simulink model "motor_pos_ctrl"  (R2023b)
settings: Solver=VariableStepAuto  StartTime=0.0  StopTime=1  RelTol=1e-3
InitFcn:
  | %%%%%%%%%%%%%%%%%%%%%%%%%%%%%%%%%%%%%%%%%%%%%%%%%
  | %motor parameters
  | %we dont know these yet
  | J = 1e-6; %intertia [kg * m^2]
  | Bm = 1e-6; %kinetic friction [N * m * s]
  | 
  | %from motor datasheet
  | Km = 0.011; %motor constant (back emf constant = torque constant)
  | Rw = 1.17; %motor electric resistance in ohms
  | Lw = 0.58E-3; %motor inductance in ohms
  | 
  | sample_time_s = 1e-3;
libraries: slpidlib x2
settings Model: Creator=you29  LastModifiedBy=you29

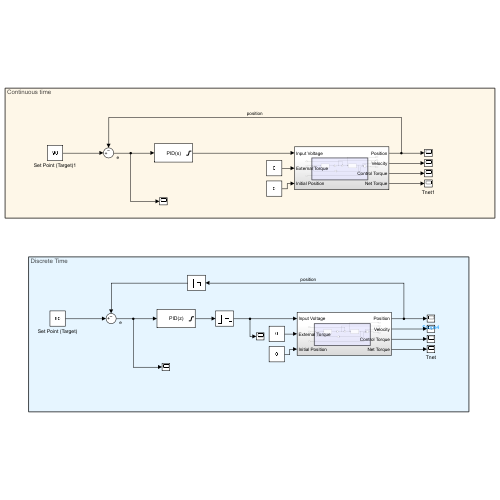
[thumbnail: Simulink's stored preview of the top-level diagram]
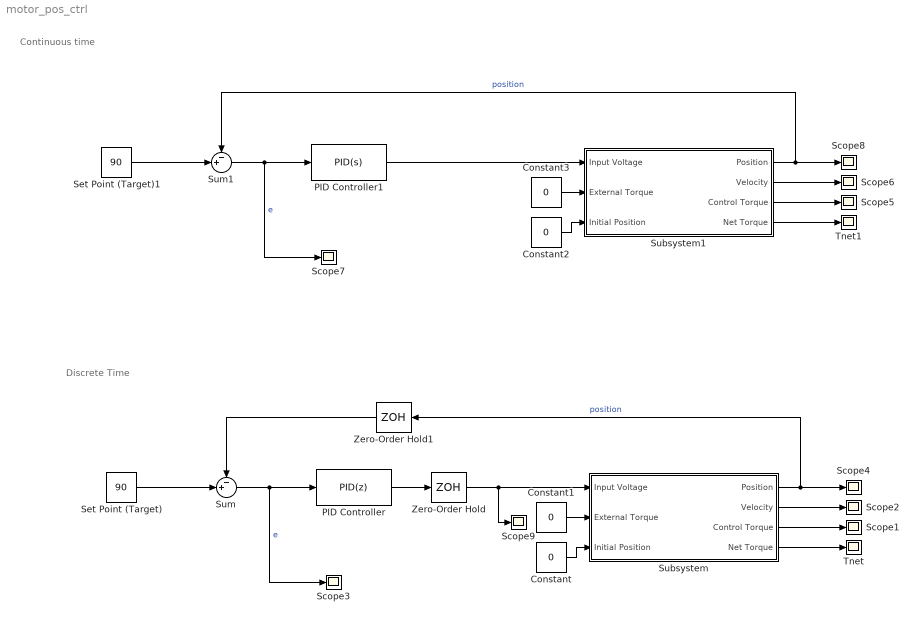
== system motor_pos_ctrl ==
  note: Continuous time
  note: Discrete Time
  Constant{,1..3} (4 alike) : Constant  Value=0
  PID Controller : slpidlib/PID Controller  Controller=PID  Form=Parallel  TimeDomain=Discrete-time  UseExternalTs=off  SampleTime=-1  IntegratorMethod=Forward Euler  FilterMethod=Forward Euler  ControllerParametersSource=internal  P=2.78055118948692  I=5  UseKiTs=off  D=0.0179888997776462  N=1  UseFilter=on  TunerSelectOption=Transfer Function Based (PID Tuner App)  InitialConditionSource=internal  InitialConditionForIntegrator=0  InitialConditionForFilter=0  DifferentiatorICPrevScaledInput=0  ExternalReset=none  TrackingMode=off  Kt=1  LimitOutput=on  SatLimitsSource=internal  UpperSaturationLimit=12  LowerSaturationLimit=-12  LinearizeAsGain=on  AntiWindupMode=none  Kb=1  LimitIntegrator=off  UpperIntegratorSaturationLimit=inf  LowerIntegratorSaturationLimit=-inf  POutMin=[]  POutMax=[]  IOutMin=[]  IOutMax=[]  DOutMin=[]  DOutMax=[]  NOutMin=[]  NOutMax=[]  SumOutMin=[]  SumOutMax=[]  SaturationOutMin=[]  SaturationOutMax=[]  PParamMin=[]  PParamMax=[]  IParamMin=[]  IParamMax=[]  DParamMin=[]  DParamMax=[]  NParamMin=[]  NParamMax=[]  KbParamMin=[]  KbParamMax=[]  KtParamMin=[]  KtParamMax=[]  KbOutMin=[]  KbOutMax=[]  KtOutMin=[]  KtOutMax=[]  IntegratorOutMin=[]  IntegratorOutMax=[]  FilterOutMin=[]  FilterOutMax=[]  SumI1OutMin=[]  SumI1OutMax=[]  SumI2OutMin=[]  SumI2OutMax=[]  SumI3OutMin=[]  SumI3OutMax=[]  SumI4OutMin=[]  SumI4OutMax=[]  SumDOutMin=[]  SumDOutMax=[]  DifferentiatorOutMin=[]  DifferentiatorOutMax=[]  FilterDiffOutCoefMin=[]  FilterDiffOutCoefMax=[]  ReciprocalOutMin=[]  ReciprocalOutMax=[]  SumDenOutMin=[]  SumDenOutMax=[]  SumNumOutMin=[]  SumNumOutMax=[]  DivideOutMin=[]  DivideOutMax=[]  UdiffTsProdOutMin=[]  UdiffTsProdOutMax=[]  NTsProdOutMin=[]  NTsProdOutMax=[]  UintegralTsProdOutMin=[]  UintegralTsProdOutMax=[]  UngainTsProdOutMin=[]  UngainTsProdOutMax=[]  ClampingZeroOutDataTypeStr=Inherit: Inherit via back propagation  ClampingZeroOutMin=[]  ClampingZeroOutMax=[]  FilterDenConstantOutDataTypeStr=Inherit: Inherit via back propagation  FilterDenConstantOutMin=[]  FilterDenConstantOutMax=[]  PCopyOutDataTypeStr=Inherit: Inherit via back propagation  PCopyOutMin=[]  PCopyOutMax=[]  NCopyOutDataTypeStr=Inherit: Inherit via back propagation  NCopyOutMin=[]  NCopyOutMax=[]  IntegratorContinuousStateAttributes=''  IntegratorStateMustResolveToSignalObject=off  IntegratorRTWStateStorageClass=Auto  FilterContinuousStateAttributes=''  FilterStateMustResolveToSignalObject=off  FilterRTWStateStorageClass=Auto  ParallelPVariant=InternalParameters  IdealPVariant=Disabled  IVariant=InternalParameters  DVariant=InternalParameters  IntegratorVariant=Discrete  SatVariant=Enabled  AWVariant=Passthrough  PCopyVariant=Disabled  TRVariant=Disabled  FdbkBlocksVariant=Forward  IdealPFdbkVariant=Disabled  SatFdbkVariant=Disabled  DerivativeFilterVariant=ForwardEulerFilter  NVariant=InternalParameters  NCopyVariant=Disabled  FilterICVariant=InternalICsFilter  IntegratorICVariant=InternalICs  ExternalResetVariant=Disabled  TRSumVariant=Passthrough  SumFdbkVariant=Disabled  SumVariant=Sum_PID  TsampFilterVariant=InternalTs  TsampNgainVariant=Passthrough  TsampIntegralVariant=Disabled_SignalSpec  ExternalSaturationOutDataTypeStr=Inherit: Same as second input
  PID Controller1 : slpidlib/PID Controller  Controller=PID  Form=Parallel  TimeDomain=Continuous-time  UseExternalTs=off  SampleTime=-1  IntegratorMethod=Forward Euler  FilterMethod=Forward Euler  ControllerParametersSource=internal  P=2.78055118948692  I=5  UseKiTs=off  D=0.0179888997776462  N=1  UseFilter=on  TunerSelectOption=Transfer Function Based (PID Tuner App)  InitialConditionSource=internal  InitialConditionForIntegrator=0  InitialConditionForFilter=0  DifferentiatorICPrevScaledInput=0  ExternalReset=none  TrackingMode=off  Kt=1  LimitOutput=on  SatLimitsSource=internal  UpperSaturationLimit=12  LowerSaturationLimit=-12  LinearizeAsGain=on  AntiWindupMode=none  Kb=1  LimitIntegrator=off  UpperIntegratorSaturationLimit=inf  LowerIntegratorSaturationLimit=-inf  POutMin=[]  POutMax=[]  IOutMin=[]  IOutMax=[]  DOutMin=[]  DOutMax=[]  NOutMin=[]  NOutMax=[]  SumOutMin=[]  SumOutMax=[]  SaturationOutMin=[]  SaturationOutMax=[]  PParamMin=[]  PParamMax=[]  IParamMin=[]  IParamMax=[]  DParamMin=[]  DParamMax=[]  NParamMin=[]  NParamMax=[]  KbParamMin=[]  KbParamMax=[]  KtParamMin=[]  KtParamMax=[]  KbOutMin=[]  KbOutMax=[]  KtOutMin=[]  KtOutMax=[]  IntegratorOutMin=[]  IntegratorOutMax=[]  FilterOutMin=[]  FilterOutMax=[]  SumI1OutMin=[]  SumI1OutMax=[]  SumI2OutMin=[]  SumI2OutMax=[]  SumI3OutMin=[]  SumI3OutMax=[]  SumI4OutMin=[]  SumI4OutMax=[]  SumDOutMin=[]  SumDOutMax=[]  DifferentiatorOutMin=[]  DifferentiatorOutMax=[]  FilterDiffOutCoefMin=[]  FilterDiffOutCoefMax=[]  ReciprocalOutMin=[]  ReciprocalOutMax=[]  SumDenOutMin=[]  SumDenOutMax=[]  SumNumOutMin=[]  SumNumOutMax=[]  DivideOutMin=[]  DivideOutMax=[]  UdiffTsProdOutMin=[]  UdiffTsProdOutMax=[]  NTsProdOutMin=[]  NTsProdOutMax=[]  UintegralTsProdOutMin=[]  UintegralTsProdOutMax=[]  UngainTsProdOutMin=[]  UngainTsProdOutMax=[]  ClampingZeroOutDataTypeStr=Inherit: Inherit via back propagation  ClampingZeroOutMin=[]  ClampingZeroOutMax=[]  FilterDenConstantOutDataTypeStr=Inherit: Inherit via back propagation  FilterDenConstantOutMin=[]  FilterDenConstantOutMax=[]  PCopyOutDataTypeStr=Inherit: Inherit via back propagation  PCopyOutMin=[]  PCopyOutMax=[]  NCopyOutDataTypeStr=Inherit: Inherit via back propagation  NCopyOutMin=[]  NCopyOutMax=[]  IntegratorContinuousStateAttributes=''  IntegratorStateMustResolveToSignalObject=off  IntegratorRTWStateStorageClass=Auto  FilterContinuousStateAttributes=''  FilterStateMustResolveToSignalObject=off  FilterRTWStateStorageClass=Auto  ParallelPVariant=InternalParameters  IdealPVariant=Disabled  IVariant=InternalParameters  DVariant=InternalParameters  IntegratorVariant=Continuous  SatVariant=Enabled  AWVariant=Passthrough  PCopyVariant=Disabled  TRVariant=Disabled  FdbkBlocksVariant=Forward  IdealPFdbkVariant=Disabled  SatFdbkVariant=Disabled  DerivativeFilterVariant=ContFilter  NVariant=InternalParameters  NCopyVariant=Disabled  FilterICVariant=InternalICsFilter  IntegratorICVariant=InternalICs  ExternalResetVariant=Disabled  TRSumVariant=Passthrough  SumFdbkVariant=Disabled  SumVariant=Sum_PID  TsampFilterVariant=InternalTs  TsampNgainVariant=Passthrough  TsampIntegralVariant=Disabled_SignalSpec  ExternalSaturationOutDataTypeStr=Inherit: Same as second input
  Scope{1..9} (9 alike) : Scope
  Set Point (Target) : Constant  Value=90
  Set Point (Target)1 : Constant  Value=90
  Subsystem : Subsystem
  Subsystem1 : Subsystem
  Sum : Sum  Inputs=-+|
  Sum1 : Sum  Inputs=-+|
  Tnet : Scope
  Tnet1 : Scope
  Zero-Order Hold : ZeroOrderHold  SampleTime=sample_time_s
  Zero-Order Hold1 : ZeroOrderHold  SampleTime=sample_time_s
  wires:
  Constant/1 -> Subsystem/3(Initial Position)
  Subsystem/1(Position) -> Scope4/1, Zero-Order Hold1/1  "position"
  Set Point (Target)/1 -> Sum/2
  Constant1/1 -> Subsystem/2(External Torque)
  Subsystem/4(Net Torque) -> Tnet/1
  Subsystem/3(Control Torque) -> Scope1/1
  Subsystem/2(Velocity) -> Scope2/1
  Sum/1 -> Scope3/1, PID Controller/1  "e"
  PID Controller/1 -> Zero-Order Hold/1
  Zero-Order Hold/1 -> Scope9/1, Subsystem/1(Input Voltage)
  Zero-Order Hold1/1 -> Sum/1
  PID Controller1/1 -> Subsystem1/1(Input Voltage)
  Sum1/1 -> Scope7/1, PID Controller1/1  "e"
  Subsystem1/3(Control Torque) -> Scope5/1
  Subsystem1/4(Net Torque) -> Tnet1/1
  Constant3/1 -> Subsystem1/2(External Torque)
  Set Point (Target)1/1 -> Sum1/2
  Subsystem1/1(Position) -> Sum1/1, Scope8/1  "position"
  Constant2/1 -> Subsystem1/3(Initial Position)
  Subsystem1/2(Velocity) -> Scope6/1

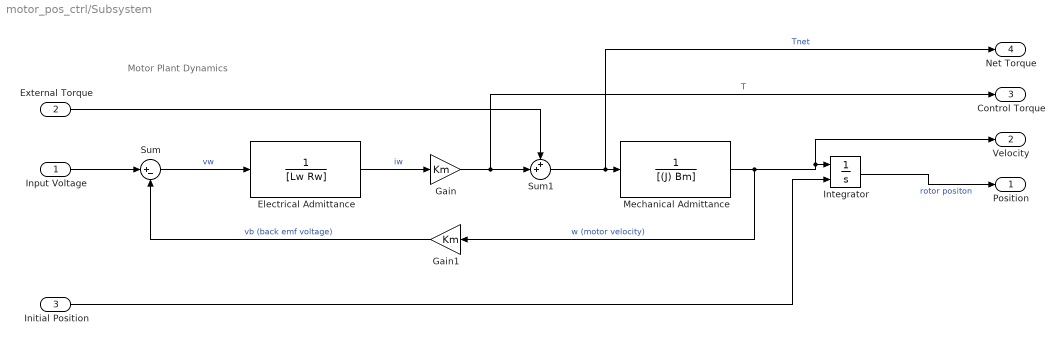
== system motor_pos_ctrl/Subsystem ==
  note: Motor Plant Dynamics
  Input Voltage : Inport
  External Torque : Inport  Port=2
  Initial Position : Inport  Port=3
  Electrical Admittance : TransferFcn  Denominator=[Lw Rw]
  Gain : Gain  Gain=Km
  Gain1 : Gain  Gain=Km
  Integrator : Integrator  InitialConditionSource=external
  Mechanical Admittance : TransferFcn  Denominator=[(J) Bm]
  Sum : Sum  Inputs=|+-
  Sum1 : Sum  Inputs=++|
  Position : Outport
  Velocity : Outport  Port=2
  Control Torque : Outport  Port=3
  Net Torque : Outport  Port=4
  wires:
  Input Voltage/1 -> Sum/1
  Mechanical Admittance/1 -> Velocity/1, Integrator/1, Gain1/1  "w (motor velocity)"
  Gain1/1 -> Sum/2  "vb (back emf voltage)"
  Integrator/1 -> Position/1  "rotor positon"
  Gain/1 -> Control Torque/1, Sum1/2  "T"
  Electrical Admittance/1 -> Gain/1  "iw"
  Sum/1 -> Electrical Admittance/1  "vw"
  Sum1/1 -> Net Torque/1, Mechanical Admittance/1  "Tnet"
  External Torque/1 -> Sum1/1
  Initial Position/1 -> Integrator/2

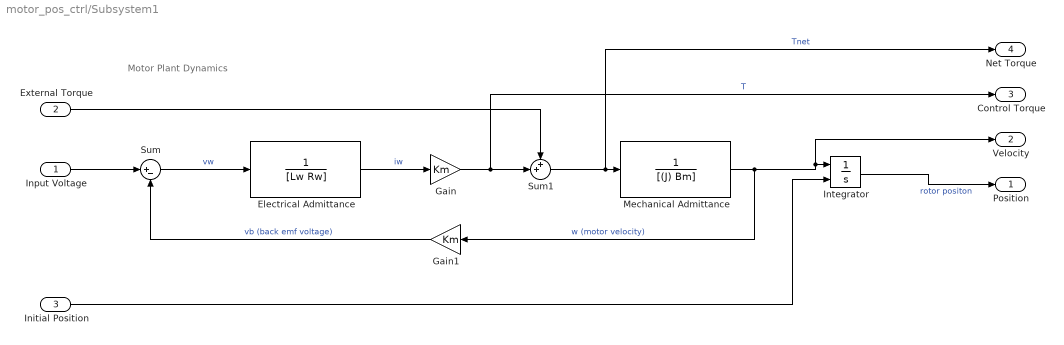
== system motor_pos_ctrl/Subsystem1 ==
  note: Motor Plant Dynamics
  Input Voltage : Inport
  External Torque : Inport  Port=2
  Initial Position : Inport  Port=3
  Electrical Admittance : TransferFcn  Denominator=[Lw Rw]
  Gain : Gain  Gain=Km
  Gain1 : Gain  Gain=Km
  Integrator : Integrator  InitialConditionSource=external
  Mechanical Admittance : TransferFcn  Denominator=[(J) Bm]
  Sum : Sum  Inputs=|+-
  Sum1 : Sum  Inputs=++|
  Position : Outport
  Velocity : Outport  Port=2
  Control Torque : Outport  Port=3
  Net Torque : Outport  Port=4
  wires:
  Input Voltage/1 -> Sum/1
  Mechanical Admittance/1 -> Velocity/1, Integrator/1, Gain1/1  "w (motor velocity)"
  Gain1/1 -> Sum/2  "vb (back emf voltage)"
  Integrator/1 -> Position/1  "rotor positon"
  Gain/1 -> Control Torque/1, Sum1/2  "T"
  Electrical Admittance/1 -> Gain/1  "iw"
  Sum/1 -> Electrical Admittance/1  "vw"
  Sum1/1 -> Net Torque/1, Mechanical Admittance/1  "Tnet"
  External Torque/1 -> Sum1/1
  Initial Position/1 -> Integrator/2
